simulink model "duel_44_my"  (R2017a)
settings: Solver=FixedStepDiscrete  StartTime=0.0  StopTime=10.0  RelTol=1e-3  EnableMultiTasking=on
settings Model: Creator=User  LastModifiedBy=Ира
settings DataIOCC: LimitDataPoints=on  SaveFormat=Array  SignalLoggingSaveFormat=ModelDataLogs
settings OptimizationCC: ExpressionDepthLimit=2147483647  InitFltsAndDblsToZero=on  LifeSpan=inf
settings DebuggingCC: SaveWithParameterizedLinksMsg=none  UnderspecifiedInitializationDetection=Classic  MergeDetectMultiDrivingBlocksExec=none  SolverPrmCheckMsg=warning  MultiTaskDSMMsg=warning  MultiTaskCondExecSysMsg=none  FcnCallInpInsideContextMsg=warning  StateNameClashWarn=warning  SFUnexpectedBacktrackingDiag=warning  SFNoUnconditionalDefaultTransitionDiag=warning  SFExecutionAtInitializationDiag=none
settings HardwareCC: ProdBitPerPointer=32  ProdBitPerSizeT=32  ProdBitPerPtrDiffT=32  ProdLargestAtomicFloat=None  ProdIntDivRoundTo=Undefined  ProdEndianess=Unspecified  ProdWordSize=32  ProdHWDeviceType=32-bit Generic  TargetBitPerPointer=64  TargetBitPerSizeT=64  TargetBitPerPtrDiffT=64  TargetLongLongMode=on  TargetIntDivRoundTo=Zero  TargetEndianess=LittleEndian  TargetWordSize=64  TargetHWDeviceType=MATLAB Host  ProdEqTarget=off
settings ModelReferenceCC: PropagateSignalLabelsOutOfModel=off
settings SFSimCC: SimParseCustomCode=off
settings GRTTargetCC: TargetLangStandard=C89/C90 (ANSI)  CombineOutputUpdateFcns=off  GRTInterface=on
settings ConfigComp: CovMetricSettings=dw  CovHtmlReporting=on  CovSaveCumulativeToWorkspaceVar=on  CovSaveSingleToWorkspaceVar=on  CovExternalEMLEnable=off

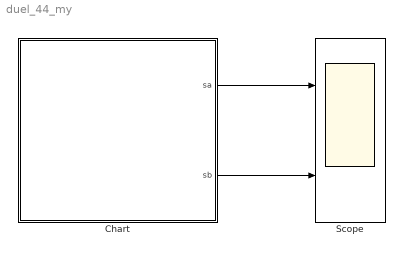
== system duel_44_my ==
  Chart : Stateflow chart  TreatAsAtomicUnit=on
  Scope : Scope  NumInputPorts=2
  wires:
  Chart/1(sa) -> Scope/1
  Chart/2(sb) -> Scope/2

== stateflow chart duel_44_my/Chart ==
  settings: updateMethod=DISCRETE  sampleTime=Ts
  state B4 [parallel]
    settings: executionOrder=1
    state life_B/
      state victory_B/
        entry: send(attack_b);
      state B_1/
        entry: bt1=t+ml('pro(LB1)');
      state B_2/
        entry: bt2=t+ml('pro(LB2)');
        k=ml('res(na0)'); ml.na0[k]=2;
      state B_3/
        entry: bt3=t+ml('pro(LB3)');
        during: p2=ml('rand');
      B4.life_B.victory_B -> B4.life_B.B_2 : [ml('sum(na0)')>0]
      (junction 171) -> B4.life_B.victory_B [order 1] : [p2<ml.pb]/ml.na0[k]=0;
      B4.life_B.B_1 -> B4.life_B.B_2 : [t>bt1]
      B4.life_B.B_3 -> (junction 171) : [t>bt3]
      (junction 171) -> B4.life_B.B_3 [order 2] : [p2>=ml.pb]/bt3=t+1;
      B4.life_B.B_2 -> B4.life_B.B_3 : [t>bt2]
    state death_B/
    (default) -> B4.life_B.B_1
    B4.life_B -> B4.death_B : attack_a[ml.nb0[4]==0]
  state A1 [parallel]
    settings: executionOrder=2
    state life_A/
      state A_1/
        entry: at1=t+ml('pro(LA1)');
      state victory_A/
        entry: send(attack_a);
      state A_2/
        entry:  at2=t+ml('pro(LA2)');
        k=ml('res(nb0)');ml.nb0[k]=2;
      state A_3/
        entry: at3=t+ml('pro(LA3)');
        during: p1=ml('rand');
      A1.life_A.victory_A -> A1.life_A.A_2 : [ml('sum(nb0)')>0]
      (junction 164) -> A1.life_A.victory_A [order 1] : [p1<ml.pa]/ml.nb0[k]=0;
      A1.life_A.A_1 -> A1.life_A.A_2 : [t>at1]
      A1.life_A.A_2 -> A1.life_A.A_3 : [t>at2]
      A1.life_A.A_3 -> (junction 164) : [t>at3]
      (junction 164) -> A1.life_A.A_3 [order 2] : [p1>=ml.pa]/at3=t+1;
    state death_A/
    (default) -> A1.life_A.A_1
    A1.life_A -> A1.death_A : attack_b[ml.na0[1]==0]
  state B1 [parallel]
    settings: executionOrder=3
    state life_B/
      state victory_B/
        entry: send(attack_b);
      state B_1/
        entry: bt1=t+ml('pro(LB1)');
      state B_2/
        entry: bt2=t+ml('pro(LB2)');
        k=ml('res(na0)'); ml.na0[k]=2;
      state B_3/
        entry: bt3=t+ml('pro(LB3)');
        during: p2=ml('rand');
      B1.life_B.victory_B -> B1.life_B.B_2 : [ml('sum(na0)')>0]
      (junction 167) -> B1.life_B.victory_B [order 1] : [p2<ml.pb]/ml.na0[k]=0;
      B1.life_B.B_1 -> B1.life_B.B_2 : [t>bt1]
      B1.life_B.B_3 -> (junction 167) : [t>bt3]
      (junction 167) -> B1.life_B.B_3 [order 2] : [p2>=ml.pb]/bt3=t+1;
      B1.life_B.B_2 -> B1.life_B.B_3 : [t>bt2]
    state death_B/
    (default) -> B1.life_B.B_1
    B1.life_B -> B1.death_B : attack_a[ml.nb0[1]==0]
  state B5 [parallel]
    settings: executionOrder=4
    state life_B/
      state victory_B/
        entry: send(attack_b);
      state B_1/
        entry: bt1=t+ml('pro(LB1)');
      state B_2/
        entry: bt2=t+ml('pro(LB2)');
        k=ml('res(na0)'); ml.na0[k]=2;
      state B_3/
        entry: bt3=t+ml('pro(LB3)');
        during: p2=ml('rand');
      B5.life_B.victory_B -> B5.life_B.B_2 : [ml('sum(na0)')>0]
      (junction 207) -> B5.life_B.victory_B [order 1] : [p2<ml.pb]/ml.na0[k]=0;
      B5.life_B.B_1 -> B5.life_B.B_2 : [t>bt1]
      B5.life_B.B_3 -> (junction 207) : [t>bt3]
      (junction 207) -> B5.life_B.B_3 [order 2] : [p2>=ml.pb]/bt3=t+1;
      B5.life_B.B_2 -> B5.life_B.B_3 : [t>bt2]
    state death_B/
    (default) -> B5.life_B.B_1
    B5.life_B -> B5.death_B : attack_a[ml.nb0[5]==0]
  state A2 [parallel]
    settings: executionOrder=5
    state life_A/
      state A_1/
        entry: at1=t+ml('pro(LA1)');
      state victory_A/
        entry: send(attack_a);
      state A_2/
        entry:  at2=t+ml('pro(LA2)');
        k=ml('res(nb0)');ml.nb0[k]=2;
      state A_3/
        entry: at3=t+ml('pro(LA3)');
        during: p1=ml('rand');
      A2.life_A.victory_A -> A2.life_A.A_2 : [ml('sum(nb0)')>0]
      (junction 165) -> A2.life_A.victory_A [order 1] : [p1<ml.pa]/ml.nb0[k]=0;
      A2.life_A.A_1 -> A2.life_A.A_2 : [t>at1]
      A2.life_A.A_2 -> A2.life_A.A_3 : [t>at2]
      A2.life_A.A_3 -> (junction 165) : [t>at3]
      (junction 165) -> A2.life_A.A_3 [order 2] : [p1>=ml.pa]/at3=t+1;
    state death_A/
    (default) -> A2.life_A.A_1
    A2.life_A -> A2.death_A : attack_b[ml.na0[2]==0]
  state B2 [parallel]
    settings: executionOrder=6
    state life_B/
      state victory_B/
        entry: send(attack_b);
      state B_1/
        entry: bt1=t+ml('pro(LB1)');
      state B_2/
        entry: bt2=t+ml('pro(LB2)');
        k=ml('res(na0)'); ml.na0[k]=2;
      state B_3/
        entry: bt3=t+ml('pro(LB3)');
        during: p2=ml('rand');
      B2.life_B.victory_B -> B2.life_B.B_2 : [ml('sum(na0)')>0]
      (junction 166) -> B2.life_B.victory_B [order 1] : [p2<ml.pb]/ml.na0[k]=0;
      B2.life_B.B_1 -> B2.life_B.B_2 : [t>bt1]
      (junction 166) -> B2.life_B.B_3 [order 2] : [p2>=ml.pb]/bt3=t+1;
      B2.life_B.B_3 -> (junction 166) : [t>bt3]
      B2.life_B.B_2 -> B2.life_B.B_3 : [t>bt2]
    state death_B/
    (default) -> B2.life_B.B_1
    B2.life_B -> B2.death_B : attack_a[ml.nb0[2]==0]
  state SUM [parallel]
    settings: executionOrder=7
    state sum/
      entry: sa=ml.NA; sb=ml.NB;
      on attack_b: sa=ml('sum(round(na0/2))');
      on attack_a: sb=ml('sum(round(nb0/2))');
  state B6 [parallel]
    settings: executionOrder=8
    state life_B/
      state victory_B/
        entry: send(attack_b);
      state B_1/
        entry: bt1=t+ml('pro(LB1)');
      state B_2/
        entry: bt2=t+ml('pro(LB2)');
        k=ml('res(na0)'); ml.na0[k]=2;
      state B_3/
        entry: bt3=t+ml('pro(LB3)');
        during: p2=ml('rand');
      B6.life_B.victory_B -> B6.life_B.B_2 : [ml('sum(na0)')>0]
      (junction 234) -> B6.life_B.victory_B [order 1] : [p2<ml.pb]/ml.na0[k]=0;
      B6.life_B.B_1 -> B6.life_B.B_2 : [t>bt1]
      B6.life_B.B_3 -> (junction 234) : [t>bt3]
      (junction 234) -> B6.life_B.B_3 [order 2] : [p2>=ml.pb]/bt3=t+1;
      B6.life_B.B_2 -> B6.life_B.B_3 : [t>bt2]
    state death_B/
    (default) -> B6.life_B.B_1
    B6.life_B -> B6.death_B : attack_a[ml.nb0[6 ]==0]
  state B3 [parallel]
    settings: executionOrder=9
    state life_B/
      state victory_B/
        entry: send(attack_b);
      state B_1/
        entry: bt1=t+ml('pro(LB1)');
      state B_2/
        entry: bt2=t+ml('pro(LB2)');
        k=ml('res(na0)'); ml.na0[k]=2;
      state B_3/
        entry: bt3=t+ml('pro(LB3)');
        during: p2=ml('rand');
      B3.life_B.victory_B -> B3.life_B.B_2 : [ml('sum(na0)')>0]
      (junction 170) -> B3.life_B.victory_B [order 1] : [p2<ml.pb]/ml.na0[k]=0;
      B3.life_B.B_1 -> B3.life_B.B_2 : [t>bt1]
      B3.life_B.B_3 -> (junction 170) : [t>bt3]
      (junction 170) -> B3.life_B.B_3 [order 2] : [p2>=ml.pb]/bt3=t+1;
      B3.life_B.B_2 -> B3.life_B.B_3 : [t>bt2]
    state death_B/
    (default) -> B3.life_B.B_1
    B3.life_B -> B3.death_B : attack_a[ml.nb0[3]==0]
  state B7 [parallel]
    settings: executionOrder=10
    state life_B/
      state victory_B/
        entry: send(attack_b);
      state B_1/
        entry: bt1=t+ml('pro(LB1)');
      state B_2/
        entry: bt2=t+ml('pro(LB2)');
        k=ml('res(na0)'); ml.na0[k]=2;
      state B_3/
        entry: bt3=t+ml('pro(LB3)');
        during: p2=ml('rand');
      B7.life_B.victory_B -> B7.life_B.B_2 : [ml('sum(na0)')>0]
      (junction 255) -> B7.life_B.victory_B [order 1] : [p2<ml.pb]/ml.na0[k]=0;
      B7.life_B.B_1 -> B7.life_B.B_2 : [t>bt1]
      B7.life_B.B_3 -> (junction 255) : [t>bt3]
      (junction 255) -> B7.life_B.B_3 [order 2] : [p2>=ml.pb]/bt3=t+1;
      B7.life_B.B_2 -> B7.life_B.B_3 : [t>bt2]
    state death_B/
    (default) -> B7.life_B.B_1
    B7.life_B -> B7.death_B : attack_a[ml.nb0[7]==0]
  (default) -> sum
  data: k local double; p2 local double; bt1 local double; bt2 local double; bt3 local double; at2 local double; p1 local double; at1 local double; k local double; at3 local double; k local double; p2 local double; bt1 local double; bt2 local double; bt3 local double; k local double; p2 local double; bt1 local double; bt2 local double; bt3 local double; at2 local double; p1 local double; at1 local double; k local double; at3 local double; bt1 local double; bt2 local double; bt3 local double; k local double; p2 local double; k local double; p2 local double; bt1 local double; bt2 local double; bt3 local double; k local double; p2 local double; bt1 local double; bt2 local double; bt3 local double; k local double; p2 local double; bt1 local double; bt2 local double; bt3 local double; sa output double; sb output double
  events: attack_a local EITHER_EDGE_EVENT; attack_b local EITHER_EDGE_EVENT
